simulink model "P702_NI_SoftECU"  (R2019a)
settings: Solver=ode1  StartTime=0.0  StopTime=Inf  FixedStep=0.001  RelTol=1e-3  EnableMultiTasking=on
PreLoadFcn:
  | run '.\VeriStand_BlockSet\NIVeriStandAddPaths.m'
undefined symbols (not defined in the file or in its folder): magnitude
libraries: simulink x83, simulink_extras x1
(part 44 of 76)

== system P702_NI_SoftECU/Input/GWM-SCCM//PDB//RCM//GSM/Other_GWMTx/ActiveFrontStrg_Stat_FD1 ==
  Bus_Sig : BusCreator  Inputs=5
  Counter Limited1 : simulink/Sources/Counter Limited  uplimit=15  tsamp=0.01
  Data Type Conversion1 : DataTypeConversion  OutDataTypeStr=uint8
  SteWhlBrkAnActl_No_Cnt : S-Function  Priority=1  Commented=on  FunctionName=NIVeriStandIO  Parameters=width dtype portnum stime stype btype  SFunctionDeploymentMode=off  EnableBusSupport=off  mask(NI VeriStand Inport){portnum=1, width=-1, stime=-1, dtype=auto, stype=auto, btype=1}
      mask prompts: portnum "Port number:"; width "Port dimensions (-1 for dynamically sized):"; stime "Sample time (-1 for inherited):"; dtype "Data type:"; stype "Signal type:"; btype "Block type:"
      mask help: Use this inport on any level of nested subsystems to allow NI VeriStand software to map signals to it.
      mask init:
      | NIVeriStandIO_init;
      settings: CopyFcn=NIVeriStand_MDL_functions('', 'IO_copy');  DeleteFcn=NIVeriStand_MDL_functions('', 'IO_delete');  MoveFcn=set_param(gcb, 'Mask', 'on');
      mask Callback portnum: NIVeriStand_MDL_functions('', 'IO_setportnum');
      mask TypeOptions dtype: auto | double | single | int8 | uint8 | int16 | uint16 | int32 | uint32 | boolean
      mask Callback dtype: NIVeriStand_MDL_functions('', 'IO_booleansignal');
      mask TypeOptions stype: auto | real | complex
      mask Display:
      | patch([-x x], [-y y], [.90980 .81960 .32156]);
      | plot([xrad -x x xrad], [yrad -y y yrad]);
      | fprintf('NI In%d', portnum);
  SteWhlBrkAnActl_No_Cnt_old_Debug : S-Function  Priority=1  FunctionName=NIVeriStandIO  Parameters=width dtype portnum stime stype btype  SFunctionDeploymentMode=off  EnableBusSupport=off  mask(NI VeriStand Outport){portnum=1, width=-1, stime=-1, dtype=auto, stype=auto, btype=0}
      mask prompts: portnum "Port number:"; width "Port dimensions (-1 for dynamically sized):"; stime "Sample time (-1 for inherited):"; dtype "Data type:"; stype "Signal type:"; btype "Block type:"
      mask help: Use this outport on any level of nested subsystems to allow NI VeriStand software to map signals to it.
      mask init:
      | NIVeriStandIO_init;
      settings: CopyFcn=NIVeriStand_MDL_functions('', 'IO_copy');  DeleteFcn=NIVeriStand_MDL_functions('', 'IO_delete');  MoveFcn=set_param(gcb, 'Mask', 'on');
      mask Callback portnum: NIVeriStand_MDL_functions('', 'IO_setportnum');
      mask TypeOptions dtype: auto | double | single | int8 | uint8 | int16 | uint16 | int32 | uint32 | boolean
      mask Callback dtype: NIVeriStand_MDL_functions('', 'IO_booleansignal');
      mask TypeOptions stype: auto | real | complex
      mask Display:
      | patch([-x x], [-y y], [.90980 .81960 .32156]);
      | plot([xrad -x x xrad], [yrad -y y yrad]);
      | fprintf('NI Out%d', portnum);
  SteWhlBrkAnActl_No_Cs : S-Function  Priority=1  FunctionName=NIVeriStandIO  Parameters=width dtype portnum stime stype btype  SFunctionDeploymentMode=off  EnableBusSupport=off  mask(NI VeriStand Inport){portnum=1, width=-1, stime=-1, dtype=auto, stype=auto, btype=1}
      mask prompts: portnum "Port number:"; width "Port dimensions (-1 for dynamically sized):"; stime "Sample time (-1 for inherited):"; dtype "Data type:"; stype "Signal type:"; btype "Block type:"
      mask help: Use this inport on any level of nested subsystems to allow NI VeriStand software to map signals to it.
      mask init:
      | NIVeriStandIO_init;
      settings: CopyFcn=NIVeriStand_MDL_functions('', 'IO_copy');  DeleteFcn=NIVeriStand_MDL_functions('', 'IO_delete');  MoveFcn=set_param(gcb, 'Mask', 'on');
      mask Callback portnum: NIVeriStand_MDL_functions('', 'IO_setportnum');
      mask TypeOptions dtype: auto | double | single | int8 | uint8 | int16 | uint16 | int32 | uint32 | boolean
      mask Callback dtype: NIVeriStand_MDL_functions('', 'IO_booleansignal');
      mask TypeOptions stype: auto | real | complex
      mask Display:
      | patch([-x x], [-y y], [.90980 .81960 .32156]);
      | plot([xrad -x x xrad], [yrad -y y yrad]);
      | fprintf('NI In%d', portnum);
  SteWhlBrkOffst_An_Actl : S-Function  Priority=2  FunctionName=NIVeriStandIO  Parameters=width dtype portnum stime stype btype  SFunctionDeploymentMode=off  EnableBusSupport=off  mask(NI VeriStand Inport){portnum=2, width=-1, stime=-1, dtype=auto, stype=auto, btype=1}
      mask prompts: portnum "Port number:"; width "Port dimensions (-1 for dynamically sized):"; stime "Sample time (-1 for inherited):"; dtype "Data type:"; stype "Signal type:"; btype "Block type:"
      mask help: Use this inport on any level of nested subsystems to allow NI VeriStand software to map signals to it.
      mask init:
      | NIVeriStandIO_init;
      settings: CopyFcn=NIVeriStand_MDL_functions('', 'IO_copy');  DeleteFcn=NIVeriStand_MDL_functions('', 'IO_delete');  MoveFcn=set_param(gcb, 'Mask', 'on');
      mask Callback portnum: NIVeriStand_MDL_functions('', 'IO_setportnum');
      mask TypeOptions dtype: auto | double | single | int8 | uint8 | int16 | uint16 | int32 | uint32 | boolean
      mask Callback dtype: NIVeriStand_MDL_functions('', 'IO_booleansignal');
      mask TypeOptions stype: auto | real | complex
      mask Display:
      | patch([-x x], [-y y], [.90980 .81960 .32156]);
      | plot([xrad -x x xrad], [yrad -y y yrad]);
      | fprintf('NI In%d', portnum);
  SteWhlOffstRq_D_Stat : S-Function  Priority=3  FunctionName=NIVeriStandIO  Parameters=width dtype portnum stime stype btype  SFunctionDeploymentMode=off  EnableBusSupport=off  mask(NI VeriStand Inport){portnum=3, width=-1, stime=-1, dtype=auto, stype=auto, btype=1}
      mask prompts: portnum "Port number:"; width "Port dimensions (-1 for dynamically sized):"; stime "Sample time (-1 for inherited):"; dtype "Data type:"; stype "Signal type:"; btype "Block type:"
      mask help: Use this inport on any level of nested subsystems to allow NI VeriStand software to map signals to it.
      mask init:
      | NIVeriStandIO_init;
      settings: CopyFcn=NIVeriStand_MDL_functions('', 'IO_copy');  DeleteFcn=NIVeriStand_MDL_functions('', 'IO_delete');  MoveFcn=set_param(gcb, 'Mask', 'on');
      mask Callback portnum: NIVeriStand_MDL_functions('', 'IO_setportnum');
      mask TypeOptions dtype: auto | double | single | int8 | uint8 | int16 | uint16 | int32 | uint32 | boolean
      mask Callback dtype: NIVeriStand_MDL_functions('', 'IO_booleansignal');
      mask TypeOptions stype: auto | real | complex
      mask Display:
      | patch([-x x], [-y y], [.90980 .81960 .32156]);
      | plot([xrad -x x xrad], [yrad -y y yrad]);
      | fprintf('NI In%d', portnum);
  SteWhlOffst_An_TotActl : S-Function  Priority=4  FunctionName=NIVeriStandIO  Parameters=width dtype portnum stime stype btype  SFunctionDeploymentMode=off  EnableBusSupport=off  mask(NI VeriStand Inport){portnum=4, width=-1, stime=-1, dtype=auto, stype=auto, btype=1}
      mask prompts: portnum "Port number:"; width "Port dimensions (-1 for dynamically sized):"; stime "Sample time (-1 for inherited):"; dtype "Data type:"; stype "Signal type:"; btype "Block type:"
      mask help: Use this inport on any level of nested subsystems to allow NI VeriStand software to map signals to it.
      mask init:
      | NIVeriStandIO_init;
      settings: CopyFcn=NIVeriStand_MDL_functions('', 'IO_copy');  DeleteFcn=NIVeriStand_MDL_functions('', 'IO_delete');  MoveFcn=set_param(gcb, 'Mask', 'on');
      mask Callback portnum: NIVeriStand_MDL_functions('', 'IO_setportnum');
      mask TypeOptions dtype: auto | double | single | int8 | uint8 | int16 | uint16 | int32 | uint32 | boolean
      mask Callback dtype: NIVeriStand_MDL_functions('', 'IO_booleansignal');
      mask TypeOptions stype: auto | real | complex
      mask Display:
      | patch([-x x], [-y y], [.90980 .81960 .32156]);
      | plot([xrad -x x xrad], [yrad -y y yrad]);
      | fprintf('NI In%d', portnum);
  ActiveFrontStrg_Stat_FD1_89 : Outport
  wires:
  Bus_Sig/1 -> ActiveFrontStrg_Stat_FD1_89/1  "ActiveFrontStrg_Stat_FD1_89"
  SteWhlBrkAnActl_No_Cs/1 -> Bus_Sig/2  "SteWhlBrkAnActl_No_Cs"
  SteWhlBrkOffst_An_Actl/1 -> Bus_Sig/3  "SteWhlBrkOffst_An_Actl"
  SteWhlOffstRq_D_Stat/1 -> Bus_Sig/4  "SteWhlOffstRq_D_Stat"
  SteWhlOffst_An_TotActl/1 -> Bus_Sig/5  "SteWhlOffst_An_TotActl"
  Counter Limited1/1 -> Data Type Conversion1/1
  Data Type Conversion1/1 -> SteWhlBrkAnActl_No_Cnt_old_Debug/1, Bus_Sig/1  "SteWhlBrkAnActl_No_Cnt"

== system P702_NI_SoftECU/Input/GWM-SCCM//PDB//RCM//GSM/Other_GWMTx/AllTerrainControlData_FD1 ==
  Bus_Sig : BusCreator  Inputs=4
  SelDrvMdeCnt_D_Stat : S-Function  Priority=1  FunctionName=NIVeriStandIO  Parameters=width dtype portnum stime stype btype  SFunctionDeploymentMode=off  EnableBusSupport=off  mask(NI VeriStand Inport){portnum=1, width=-1, stime=-1, dtype=auto, stype=auto, btype=1}
      mask prompts: portnum "Port number:"; width "Port dimensions (-1 for dynamically sized):"; stime "Sample time (-1 for inherited):"; dtype "Data type:"; stype "Signal type:"; btype "Block type:"
      mask help: Use this inport on any level of nested subsystems to allow NI VeriStand software to map signals to it.
      mask init:
      | NIVeriStandIO_init;
      settings: CopyFcn=NIVeriStand_MDL_functions('', 'IO_copy');  DeleteFcn=NIVeriStand_MDL_functions('', 'IO_delete');  MoveFcn=set_param(gcb, 'Mask', 'on');
      mask Callback portnum: NIVeriStand_MDL_functions('', 'IO_setportnum');
      mask TypeOptions dtype: auto | double | single | int8 | uint8 | int16 | uint16 | int32 | uint32 | boolean
      mask Callback dtype: NIVeriStand_MDL_functions('', 'IO_booleansignal');
      mask TypeOptions stype: auto | real | complex
      mask Display:
      | patch([-x x], [-y y], [.90980 .81960 .32156]);
      | plot([xrad -x x xrad], [yrad -y y yrad]);
      | fprintf('NI In%d', portnum);
  SelDrvMdeSwtchOk_D_Stat : S-Function  Priority=2  FunctionName=NIVeriStandIO  Parameters=width dtype portnum stime stype btype  SFunctionDeploymentMode=off  EnableBusSupport=off  mask(NI VeriStand Inport){portnum=2, width=-1, stime=-1, dtype=auto, stype=auto, btype=1}
      mask prompts: portnum "Port number:"; width "Port dimensions (-1 for dynamically sized):"; stime "Sample time (-1 for inherited):"; dtype "Data type:"; stype "Signal type:"; btype "Block type:"
      mask help: Use this inport on any level of nested subsystems to allow NI VeriStand software to map signals to it.
      mask init:
      | NIVeriStandIO_init;
      settings: CopyFcn=NIVeriStand_MDL_functions('', 'IO_copy');  DeleteFcn=NIVeriStand_MDL_functions('', 'IO_delete');  MoveFcn=set_param(gcb, 'Mask', 'on');
      mask Callback portnum: NIVeriStand_MDL_functions('', 'IO_setportnum');
      mask TypeOptions dtype: auto | double | single | int8 | uint8 | int16 | uint16 | int32 | uint32 | boolean
      mask Callback dtype: NIVeriStand_MDL_functions('', 'IO_booleansignal');
      mask TypeOptions stype: auto | real | complex
      mask Display:
      | patch([-x x], [-y y], [.90980 .81960 .32156]);
      | plot([xrad -x x xrad], [yrad -y y yrad]);
      | fprintf('NI In%d', portnum);
  SelDrvMdeSwtch_D_Stat : S-Function  Priority=3  FunctionName=NIVeriStandIO  Parameters=width dtype portnum stime stype btype  SFunctionDeploymentMode=off  EnableBusSupport=off  mask(NI VeriStand Inport){portnum=3, width=-1, stime=-1, dtype=auto, stype=auto, btype=1}
      mask prompts: portnum "Port number:"; width "Port dimensions (-1 for dynamically sized):"; stime "Sample time (-1 for inherited):"; dtype "Data type:"; stype "Signal type:"; btype "Block type:"
      mask help: Use this inport on any level of nested subsystems to allow NI VeriStand software to map signals to it.
      mask init:
      | NIVeriStandIO_init;
      settings: CopyFcn=NIVeriStand_MDL_functions('', 'IO_copy');  DeleteFcn=NIVeriStand_MDL_functions('', 'IO_delete');  MoveFcn=set_param(gcb, 'Mask', 'on');
      mask Callback portnum: NIVeriStand_MDL_functions('', 'IO_setportnum');
      mask TypeOptions dtype: auto | double | single | int8 | uint8 | int16 | uint16 | int32 | uint32 | boolean
      mask Callback dtype: NIVeriStand_MDL_functions('', 'IO_booleansignal');
      mask TypeOptions stype: auto | real | complex
      mask Display:
      | patch([-x x], [-y y], [.90980 .81960 .32156]);
      | plot([xrad -x x xrad], [yrad -y y yrad]);
      | fprintf('NI In%d', portnum);
  SelDrvMdeSwtch_No_Actl : S-Function  Priority=4  FunctionName=NIVeriStandIO  Parameters=width dtype portnum stime stype btype  SFunctionDeploymentMode=off  EnableBusSupport=off  mask(NI VeriStand Inport){portnum=4, width=-1, stime=-1, dtype=auto, stype=auto, btype=1}
      mask prompts: portnum "Port number:"; width "Port dimensions (-1 for dynamically sized):"; stime "Sample time (-1 for inherited):"; dtype "Data type:"; stype "Signal type:"; btype "Block type:"
      mask help: Use this inport on any level of nested subsystems to allow NI VeriStand software to map signals to it.
      mask init:
      | NIVeriStandIO_init;
      settings: CopyFcn=NIVeriStand_MDL_functions('', 'IO_copy');  DeleteFcn=NIVeriStand_MDL_functions('', 'IO_delete');  MoveFcn=set_param(gcb, 'Mask', 'on');
      mask Callback portnum: NIVeriStand_MDL_functions('', 'IO_setportnum');
      mask TypeOptions dtype: auto | double | single | int8 | uint8 | int16 | uint16 | int32 | uint32 | boolean
      mask Callback dtype: NIVeriStand_MDL_functions('', 'IO_booleansignal');
      mask TypeOptions stype: auto | real | complex
      mask Display:
      | patch([-x x], [-y y], [.90980 .81960 .32156]);
      | plot([xrad -x x xrad], [yrad -y y yrad]);
      | fprintf('NI In%d', portnum);
  AllTerrainControlData_FD1_461 : Outport
  wires:
  Bus_Sig/1 -> AllTerrainControlData_FD1_461/1  "AllTerrainControlData_FD1_461"
  SelDrvMdeCnt_D_Stat/1 -> Bus_Sig/1  "SelDrvMdeCnt_D_Stat"
  SelDrvMdeSwtchOk_D_Stat/1 -> Bus_Sig/2  "SelDrvMdeSwtchOk_D_Stat"
  SelDrvMdeSwtch_D_Stat/1 -> Bus_Sig/3  "SelDrvMdeSwtch_D_Stat"
  SelDrvMdeSwtch_No_Actl/1 -> Bus_Sig/4  "SelDrvMdeSwtch_No_Actl"

== system P702_NI_SoftECU/Input/GWM-SCCM//PDB//RCM//GSM/Other_GWMTx/All_Terrain_Data_FD1 ==
  Bus_Sig : BusCreator  Inputs=2
  TerrMde_D_RqDrv : Constant  Value=0
  TerrStat_D_RqDsply : Constant  Value=0
  All_Terrain_Data_FD1_481 : Outport
  wires:
  Bus_Sig/1 -> All_Terrain_Data_FD1_481/1  "All_Terrain_Data_FD1_481"
  TerrMde_D_RqDrv/1 -> Bus_Sig/1  "TerrMde_D_RqDrv"
  TerrStat_D_RqDsply/1 -> Bus_Sig/2  "TerrStat_D_RqDsply"

== system P702_NI_SoftECU/Input/GWM-SCCM//PDB//RCM//GSM/Other_GWMTx/BCM_Lamp_Stat_FD1 ==
  BrkWarnInd_B_Rq : Constant  Value=0
  Brk_Fluid_Lvl_Low : Constant  Value=0
  Bus_Sig : BusCreator  Inputs=35
  Courtesy_BSave_Stat : Constant
  Courtesy_Delay_Status : Constant  Value=0
  CrnrLghtLeft_Pc_Rq : Constant  Value=0
  CrnrLghtRight_Pc_Rq : Constant  Value=0
  DayRnngLampOn_B_Stat : Constant  Value=0
  DrTgateLck_D_Stat : Constant  Value=0
  Dr_Courtesy_Light_Stat : Constant  Value=0
  HeadLampLoActv_B_Stat : Constant
  HeadLampLoFlOn_B_Stat : Constant
  HeadLampLoFrOn_B_Stat : Constant
  HeadLampLoOut_B_Stat : Constant  Value=0
  HeadLghtHiFdbck_D_Stat : Constant  Value=0
  HeadLghtHiOn_B_Stat : Constant  Value=0
  HeadLghtSwtch_D_Stat : Constant  Value=2
  Headlamp_On_Wrning_Cmd : Constant  Value=0
  HomeSafeLtChime_B_Rq : Constant  Value=0
  Illuminated_Entry_Stat : Constant  Value=0
  ImpactEvntFdbck_D_Stat : Constant  Value=0
  KeyInIgnWarn_B_Cmd : Constant  Value=0
  Park_Brake_Chime_Rqst : Constant  Value=0
  PerimeterAlarmChimeRq : Constant  Value=0
  Perimeter_Alarm_Status : Constant  Value=0
  PrkLght_D_Stat : Constant  Value=0
  PrkLightChime_B_Rq : Constant  Value=0
  PudLampDrv_D_Rq : Constant  Value=0
  PudLampPsngr_D_Rq : Constant  Value=0
  PudLamp_D_Rq : Constant  Value=0
  ReducedGuard_D_Stat : Constant  Value=0
  RvrseLghtOn_B_Stat : Constant  Value=0
  StopLghtOn_B_Stat : Constant  Value=0
  TrnNotInPrkChime_B_Rq : Constant  Value=0
  WndwGlbl_D_Cmd : Constant  Value=0
  WrlssAcsyChrgInhbt_B_Rq : Constant  Value=0
  BCM_Lamp_Stat_FD1_3C3 : Outport
  wires:
  Bus_Sig/1 -> BCM_Lamp_Stat_FD1_3C3/1  "BCM_Lamp_Stat_FD1_3C3"
  BrkWarnInd_B_Rq/1 -> Bus_Sig/1  "BrkWarnInd_B_Rq"
  Brk_Fluid_Lvl_Low/1 -> Bus_Sig/2  "Brk_Fluid_Lvl_Low"
  Courtesy_BSave_Stat/1 -> Bus_Sig/3  "Courtesy_BSave_Stat"
  Courtesy_Delay_Status/1 -> Bus_Sig/4  "Courtesy_Delay_Status"
  CrnrLghtLeft_Pc_Rq/1 -> Bus_Sig/5  "CrnrLghtLeft_Pc_Rq"
  CrnrLghtRight_Pc_Rq/1 -> Bus_Sig/6  "CrnrLghtRight_Pc_Rq"
  DayRnngLampOn_B_Stat/1 -> Bus_Sig/7  "DayRnngLampOn_B_Stat"
  DrTgateLck_D_Stat/1 -> Bus_Sig/8  "DrTgateLck_D_Stat"
  Dr_Courtesy_Light_Stat/1 -> Bus_Sig/9  "Dr_Courtesy_Light_Stat"
  HeadLampLoActv_B_Stat/1 -> Bus_Sig/10  "HeadLampLoActv_B_Stat"
  HeadLampLoFlOn_B_Stat/1 -> Bus_Sig/11  "HeadLampLoFlOn_B_Stat"
  HeadLampLoFrOn_B_Stat/1 -> Bus_Sig/12  "HeadLampLoFrOn_B_Stat"
  HeadLampLoOut_B_Stat/1 -> Bus_Sig/13  "HeadLampLoOut_B_Stat"
  HeadLghtHiFdbck_D_Stat/1 -> Bus_Sig/14  "HeadLghtHiFdbck_D_Stat"
  HeadLghtHiOn_B_Stat/1 -> Bus_Sig/15  "HeadLghtHiOn_B_Stat"
  HeadLghtSwtch_D_Stat/1 -> Bus_Sig/16  "HeadLghtSwtch_D_Stat"
  Headlamp_On_Wrning_Cmd/1 -> Bus_Sig/17  "Headlamp_On_Wrning_Cmd"
  HomeSafeLtChime_B_Rq/1 -> Bus_Sig/18  "HomeSafeLtChime_B_Rq"
  Illuminated_Entry_Stat/1 -> Bus_Sig/19  "Illuminated_Entry_Stat"
  ImpactEvntFdbck_D_Stat/1 -> Bus_Sig/20  "ImpactEvntFdbck_D_Stat"
  KeyInIgnWarn_B_Cmd/1 -> Bus_Sig/21  "KeyInIgnWarn_B_Cmd"
  Park_Brake_Chime_Rqst/1 -> Bus_Sig/22  "Park_Brake_Chime_Rqst"
  PerimeterAlarmChimeRq/1 -> Bus_Sig/23  "PerimeterAlarmChimeRq"
  Perimeter_Alarm_Status/1 -> Bus_Sig/24  "Perimeter_Alarm_Status"
  PrkLght_D_Stat/1 -> Bus_Sig/25  "PrkLght_D_Stat"
  PrkLightChime_B_Rq/1 -> Bus_Sig/26  "PrkLightChime_B_Rq"
  PudLampDrv_D_Rq/1 -> Bus_Sig/27  "PudLampDrv_D_Rq"
  PudLampPsngr_D_Rq/1 -> Bus_Sig/28  "PudLampPsngr_D_Rq"
  PudLamp_D_Rq/1 -> Bus_Sig/29  "PudLamp_D_Rq"
  ReducedGuard_D_Stat/1 -> Bus_Sig/30  "ReducedGuard_D_Stat"
  RvrseLghtOn_B_Stat/1 -> Bus_Sig/31  "RvrseLghtOn_B_Stat"
  StopLghtOn_B_Stat/1 -> Bus_Sig/32  "StopLghtOn_B_Stat"
  TrnNotInPrkChime_B_Rq/1 -> Bus_Sig/33  "TrnNotInPrkChime_B_Rq"
  WndwGlbl_D_Cmd/1 -> Bus_Sig/34  "WndwGlbl_D_Cmd"
  WrlssAcsyChrgInhbt_B_Rq/1 -> Bus_Sig/35  "WrlssAcsyChrgInhbt_B_Rq"

== system P702_NI_SoftECU/Input/GWM-SCCM//PDB//RCM//GSM/Other_GWMTx/BatteryCharge_Data2_FD1 ==
  Bus_Sig : BusCreator  Inputs=1
  ChrgCrdLck_D_Falt : Constant  Value=0
  BatteryCharge_Data2_FD1_45E : Outport
  wires:
  Bus_Sig/1 -> BatteryCharge_Data2_FD1_45E/1  "BatteryCharge_Data2_FD1_45E"
  ChrgCrdLck_D_Falt/1 -> Bus_Sig/1  "ChrgCrdLck_D_Falt"

== system P702_NI_SoftECU/Input/GWM-SCCM//PDB//RCM//GSM/Other_GWMTx/Battery_Mgmt_24V_FD1 ==
  BattULo24Soc_Pc_Actl : Constant  Value=0
  BattULo24State_D_Qlty : Constant
  BattULo24_Ah_DeltaRide : Constant  Value=12800
  BattULo24_B_Falt : Constant  Value=0
  BattULo24_I_Actl : Constant  Value=8192
  Bus_Sig : BusCreator  Inputs=5
  Battery_Mgmt_24V_FD1_42E : Outport
  wires:
  Bus_Sig/1 -> Battery_Mgmt_24V_FD1_42E/1  "Battery_Mgmt_24V_FD1_42E"
  BattULo24Soc_Pc_Actl/1 -> Bus_Sig/1  "BattULo24Soc_Pc_Actl"
  BattULo24State_D_Qlty/1 -> Bus_Sig/2  "BattULo24State_D_Qlty"
  BattULo24_Ah_DeltaRide/1 -> Bus_Sig/3  "BattULo24_Ah_DeltaRide"
  BattULo24_B_Falt/1 -> Bus_Sig/4  "BattULo24_B_Falt"
  BattULo24_I_Actl/1 -> Bus_Sig/5  "BattULo24_I_Actl"

== system P702_NI_SoftECU/Input/GWM-SCCM//PDB//RCM//GSM/Other_GWMTx/Battery_Mgmt_2_FD1 ==
  BattULoChrg_D_Rq : Constant  Value=0
  BattULoSrvc_T_Actl : Constant  Value=0
  Batt_Crit_SoC_B : Constant  Value=0
  Batt_Lo_SoC_B : Constant  Value=0
  Bus_Sig : BusCreator  Inputs=14
  ChargeMode : Constant  Value=0
  EngStrtInhbt_B_RqBatt : Constant  Value=0
  IdleSpeedIncrease_El : Constant  Value=0
  PeriodicElLoad_B_Stat : Constant  Value=0
  PwSysULoFalt_D_Stat : Constant  Value=0
  Shed_Drain_Eng_Off_B : Constant  Value=0
  Shed_Feature_Group_ID : Constant  Value=0
  Shed_Level_Req : Constant  Value=0
  Shed_T_Eng_Off_B : Constant  Value=0
  ULoRgenTestMde_B_Rq : Constant  Value=0
  Battery_Mgmt_2_FD1_42C : Outport
  wires:
  Bus_Sig/1 -> Battery_Mgmt_2_FD1_42C/1  "Battery_Mgmt_2_FD1_42C"
  BattULoChrg_D_Rq/1 -> Bus_Sig/1  "BattULoChrg_D_Rq"
  BattULoSrvc_T_Actl/1 -> Bus_Sig/2  "BattULoSrvc_T_Actl"
  Batt_Crit_SoC_B/1 -> Bus_Sig/3  "Batt_Crit_SoC_B"
  Batt_Lo_SoC_B/1 -> Bus_Sig/4  "Batt_Lo_SoC_B"
  ChargeMode/1 -> Bus_Sig/5  "ChargeMode"
  EngStrtInhbt_B_RqBatt/1 -> Bus_Sig/6  "EngStrtInhbt_B_RqBatt"
  IdleSpeedIncrease_El/1 -> Bus_Sig/7  "IdleSpeedIncrease_El"
  PeriodicElLoad_B_Stat/1 -> Bus_Sig/8  "PeriodicElLoad_B_Stat"
  PwSysULoFalt_D_Stat/1 -> Bus_Sig/9  "PwSysULoFalt_D_Stat"
  Shed_Drain_Eng_Off_B/1 -> Bus_Sig/10  "Shed_Drain_Eng_Off_B"
  Shed_Feature_Group_ID/1 -> Bus_Sig/11  "Shed_Feature_Group_ID"
  Shed_Level_Req/1 -> Bus_Sig/12  "Shed_Level_Req"
  Shed_T_Eng_Off_B/1 -> Bus_Sig/13  "Shed_T_Eng_Off_B"
  ULoRgenTestMde_B_Rq/1 -> Bus_Sig/14  "ULoRgenTestMde_B_Rq"

== system P702_NI_SoftECU/Input/GWM-SCCM//PDB//RCM//GSM/Other_GWMTx/Battery_Mgmt_3_FD1 ==
  BSBattQCapAh : Constant  Value=0
  BSBattQDeltaRideAh : Constant  Value=0
  BSBattSOC : Constant  Value=0
  BSFault : Constant  Value=0
  BattULo2_Te_Actl : Constant  Value=127
  BattULoChrg_URate_RqMx : Constant  Value=5
  BattULoChrg_U_RqMn : Constant  Value=0
  BattULoChrg_U_RqMx : Constant  Value=34
  BattULoState_D_Qlty : Constant  Value=0
  Bus_Sig : BusCreator  Inputs=9
  Battery_Mgmt_3_FD1_43C : Outport
  wires:
  Bus_Sig/1 -> Battery_Mgmt_3_FD1_43C/1  "Battery_Mgmt_3_FD1_43C"
  BSBattQCapAh/1 -> Bus_Sig/1  "BSBattQCapAh"
  BSBattQDeltaRideAh/1 -> Bus_Sig/2  "BSBattQDeltaRideAh"
  BSBattSOC/1 -> Bus_Sig/3  "BSBattSOC"
  BSFault/1 -> Bus_Sig/4  "BSFault"
  BattULo2_Te_Actl/1 -> Bus_Sig/5  "BattULo2_Te_Actl"
  BattULoChrg_URate_RqMx/1 -> Bus_Sig/6  "BattULoChrg_URate_RqMx"
  BattULoChrg_U_RqMn/1 -> Bus_Sig/7  "BattULoChrg_U_RqMn"
  BattULoChrg_U_RqMx/1 -> Bus_Sig/8  "BattULoChrg_U_RqMx"
  BattULoState_D_Qlty/1 -> Bus_Sig/9  "BattULoState_D_Qlty"

== system P702_NI_SoftECU/Input/GWM-SCCM//PDB//RCM//GSM/Other_GWMTx/Battery_Mgmt_4_FD1 ==
  BattULoAuxSoc_Pc_Actl : Constant  Value=95
  BattULoAux_B_Falt : Constant  Value=0
  BattULoAux_D_Qlty : Constant  Value=0
  BattULoAux_I_Actl : Constant  Value=0
  BattULoAux_U_Actl : Constant  Value=203
  BattULoCrnkBelt_U_Pred : Constant  Value=0
  BattULoCrnkStrt_U_Pred : Constant  Value=0
  Bus_Sig : BusCreator  Inputs=7
  Battery_Mgmt_4_FD1_42B : Outport
  wires:
  Bus_Sig/1 -> Battery_Mgmt_4_FD1_42B/1  "Battery_Mgmt_4_FD1_42B"
  BattULoAuxSoc_Pc_Actl/1 -> Bus_Sig/1  "BattULoAuxSoc_Pc_Actl"
  BattULoAux_B_Falt/1 -> Bus_Sig/2  "BattULoAux_B_Falt"
  BattULoAux_D_Qlty/1 -> Bus_Sig/3  "BattULoAux_D_Qlty"
  BattULoAux_I_Actl/1 -> Bus_Sig/4  "BattULoAux_I_Actl"
  BattULoAux_U_Actl/1 -> Bus_Sig/5  "BattULoAux_U_Actl"
  BattULoCrnkBelt_U_Pred/1 -> Bus_Sig/6  "BattULoCrnkBelt_U_Pred"
  BattULoCrnkStrt_U_Pred/1 -> Bus_Sig/7  "BattULoCrnkStrt_U_Pred"

== system P702_NI_SoftECU/Input/GWM-SCCM//PDB//RCM//GSM/Other_GWMTx/Battery_Traction_1_FD1 ==
  BattTracMil_D_Rq : Constant  Value=0
  BattTracOffFst_D_Actl : Constant  Value=0
  BattTracOff_B_Actl : Constant  Value=0
  BattTrac_I_Actl : Constant  Value=0
  BattTrac_U_Actl : Constant  Value=1022
  BattTrac_U_LimHi : Constant  Value=163
  BattTrac_U_LimLo : Constant  Value=88
  Bus_Sig : BusCreator  Inputs=8
  VehStrtInhbt_B_RqBatt : Constant  Value=0
  Battery_Traction_1_FD1_7A : Outport
  wires:
  Bus_Sig/1 -> Battery_Traction_1_FD1_7A/1  "Battery_Traction_1_FD1_7A"
  BattTracMil_D_Rq/1 -> Bus_Sig/1  "BattTracMil_D_Rq"
  BattTracOffFst_D_Actl/1 -> Bus_Sig/2  "BattTracOffFst_D_Actl"
  BattTracOff_B_Actl/1 -> Bus_Sig/3  "BattTracOff_B_Actl"
  BattTrac_I_Actl/1 -> Bus_Sig/4  "BattTrac_I_Actl"
  BattTrac_U_Actl/1 -> Bus_Sig/5  "BattTrac_U_Actl"
  BattTrac_U_LimHi/1 -> Bus_Sig/6  "BattTrac_U_LimHi"
  BattTrac_U_LimLo/1 -> Bus_Sig/7  "BattTrac_U_LimLo"
  VehStrtInhbt_B_RqBatt/1 -> Bus_Sig/8  "VehStrtInhbt_B_RqBatt"

== system P702_NI_SoftECU/Input/GWM-SCCM//PDB//RCM//GSM/Other_GWMTx/Battery_Traction_3_FD1 ==
  BattTracClnt_Te_Actl : Constant  Value=164
  BattTracSoc_Pc_LimHi : Constant  Value=600
  BattTracSoc_Pc_LimLo : Constant  Value=400
  BattTracSoc_Pc_MnPrtct : Constant  Value=30
  BattTracSoc_Pc_MxPrtct : Constant  Value=700
  BattTracSrvcRqd_B_Rq : Constant  Value=0
  BattTracWarnLamp_B_Rq : Constant  Value=0
  Bus_Sig : BusCreator  Inputs=7
  Battery_Traction_3_FD1_24B : Outport
  wires:
  Bus_Sig/1 -> Battery_Traction_3_FD1_24B/1  "Battery_Traction_3_FD1_24B"
  BattTracClnt_Te_Actl/1 -> Bus_Sig/1  "BattTracClnt_Te_Actl"
  BattTracSoc_Pc_LimHi/1 -> Bus_Sig/2  "BattTracSoc_Pc_LimHi"
  BattTracSoc_Pc_LimLo/1 -> Bus_Sig/3  "BattTracSoc_Pc_LimLo"
  BattTracSoc_Pc_MnPrtct/1 -> Bus_Sig/4  "BattTracSoc_Pc_MnPrtct"
  BattTracSoc_Pc_MxPrtct/1 -> Bus_Sig/5  "BattTracSoc_Pc_MxPrtct"
  BattTracSrvcRqd_B_Rq/1 -> Bus_Sig/6  "BattTracSrvcRqd_B_Rq"
  BattTracWarnLamp_B_Rq/1 -> Bus_Sig/7  "BattTracWarnLamp_B_Rq"

== system P702_NI_SoftECU/Input/GWM-SCCM//PDB//RCM//GSM/Other_GWMTx/Battery_Traction_4_FD1 ==
  BattTracDiagClr_B_Rq : Constant  Value=0
  BattTracSoc2_Pc_Actl : Constant  Value=16382
  BattTrac_Te_Actl : Constant  Value=150
  Bus_Sig : BusCreator  Inputs=3
  Battery_Traction_4_FD1_24C : Outport
  wires:
  Bus_Sig/1 -> Battery_Traction_4_FD1_24C/1  "Battery_Traction_4_FD1_24C"
  BattTracDiagClr_B_Rq/1 -> Bus_Sig/1  "BattTracDiagClr_B_Rq"
  BattTracSoc2_Pc_Actl/1 -> Bus_Sig/2  "BattTracSoc2_Pc_Actl"
  BattTrac_Te_Actl/1 -> Bus_Sig/3  "BattTrac_Te_Actl"

== system P702_NI_SoftECU/Input/GWM-SCCM//PDB//RCM//GSM/Other_GWMTx/Battery_Traction_5_FD1 ==
  BattTrac2_Pw_ChrgInst : Constant  Value=0
  BattTrac2_Pw_DchrgInst : Constant  Value=0
  BattTrac2_Pw_LimChrg : Constant  Value=0
  BattTrac2_Pw_LimDchrg : Constant  Value=0
  Bus_Sig : BusCreator  Inputs=4
  Battery_Traction_5_FD1_24D : Outport
  wires:
  Bus_Sig/1 -> Battery_Traction_5_FD1_24D/1  "Battery_Traction_5_FD1_24D"
  BattTrac2_Pw_ChrgInst/1 -> Bus_Sig/1  "BattTrac2_Pw_ChrgInst"
  BattTrac2_Pw_DchrgInst/1 -> Bus_Sig/2  "BattTrac2_Pw_DchrgInst"
  BattTrac2_Pw_LimChrg/1 -> Bus_Sig/3  "BattTrac2_Pw_LimChrg"
  BattTrac2_Pw_LimDchrg/1 -> Bus_Sig/4  "BattTrac2_Pw_LimDchrg"

== system P702_NI_SoftECU/Input/GWM-SCCM//PDB//RCM//GSM/Other_GWMTx/Battery_Traction_6_FD1 ==
  BattTracClntPmp_D_Stat : Constant  Value=0
  BattTracCnnct_D_Cmd : Constant  Value=0
  BattTracDcdcDis_B_Rq : Constant  Value=0
  BattTracDelta_Te_Actl : Constant  Value=120
  BattTracHvilOpen_B_Stat : Constant  Value=0
  Bus_Sig : BusCreator  Inputs=6
  HtrnClntPump_D_Stat : Constant  Value=0
  Battery_Traction_6_FD1_458 : Outport
  wires:
  Bus_Sig/1 -> Battery_Traction_6_FD1_458/1  "Battery_Traction_6_FD1_458"
  BattTracClntPmp_D_Stat/1 -> Bus_Sig/1  "BattTracClntPmp_D_Stat"
  BattTracCnnct_D_Cmd/1 -> Bus_Sig/2  "BattTracCnnct_D_Cmd"
  BattTracDcdcDis_B_Rq/1 -> Bus_Sig/3  "BattTracDcdcDis_B_Rq"
  BattTracDelta_Te_Actl/1 -> Bus_Sig/4  "BattTracDelta_Te_Actl"
  BattTracHvilOpen_B_Stat/1 -> Bus_Sig/5  "BattTracHvilOpen_B_Stat"
  HtrnClntPump_D_Stat/1 -> Bus_Sig/6  "HtrnClntPump_D_Stat"

== system P702_NI_SoftECU/Input/GWM-SCCM//PDB//RCM//GSM/Other_GWMTx/BodyInfo_3_FD1 ==
  Backlit_LED_Status : Constant  Value=0
  BodySrvcRqd_B_Rq : Constant  Value=0
  Bus_Sig : BusCreator  Inputs=31
  CrashEvnt_D_Stat : Constant  Value=3
  Day_Night_Status : Constant  Value=0
  Delay_Accy : Constant  Value=0
  DimmingLvlEvnt_No_Actl : Constant  Value=0
  Dimming_Lvl : Constant  Value=12
  DrStatDrvErrCnt_B_Stat : Constant  Value=0
  DrStatDrv_B_Actl : Constant  Value=0
  DrStatHood_B_Actl : Constant  Value=0
  DrStatInnrTgate_B_Actl : Constant  Value=0
  DrStatPsngr_B_Actl : Constant  Value=0
  DrStatRl_B_Actl : Constant  Value=0
  DrStatRr_B_Actl : Constant  Value=0
  DrStatTgate_B_Actl : Constant  Value=0
  FogLghtFrontOn_B_Stat : Constant  Value=0
  FogLghtRearOn_B_Stat : Constant  Value=0
  FuelPmpInhbt_B_Stat : Constant  Value=0
  IgnKeyType_D_Actl : Constant  Value=14
  Ignition_Status : Constant  Value=0
  Key_In_Ignition_Stat : Constant  Value=0
  LifeCycMde_D_Actl : Constant  Value=0
  Litval : Constant  Value=0
  Parklamp_Status : Constant
  PrkBrkActv_B_Actl : Constant  Value=0
  Remote_Start_Status : Constant  Value=0
  TurnLghtLeftOn_B_Stat : Constant  Value=0
  TurnLghtLeft_D_Rq : Constant  Value=0
  TurnLghtRightOn_B_Stat : Constant  Value=0
  TurnLghtRight_D_Rq : Constant  Value=0
  ValetMode_D_Mem : Constant  Value=0
  BodyInfo_3_FD1_3B3 : Outport
  wires:
  Bus_Sig/1 -> BodyInfo_3_FD1_3B3/1  "BodyInfo_3_FD1_3B3"
  Backlit_LED_Status/1 -> Bus_Sig/1  "Backlit_LED_Status"
  BodySrvcRqd_B_Rq/1 -> Bus_Sig/2  "BodySrvcRqd_B_Rq"
  CrashEvnt_D_Stat/1 -> Bus_Sig/3  "CrashEvnt_D_Stat"
  Day_Night_Status/1 -> Bus_Sig/4  "Day_Night_Status"
  Delay_Accy/1 -> Bus_Sig/5  "Delay_Accy"
  DimmingLvlEvnt_No_Actl/1 -> Bus_Sig/6  "DimmingLvlEvnt_No_Actl"
  Dimming_Lvl/1 -> Bus_Sig/7  "Dimming_Lvl"
  DrStatDrvErrCnt_B_Stat/1 -> Bus_Sig/8  "DrStatDrvErrCnt_B_Stat"
  DrStatDrv_B_Actl/1 -> Bus_Sig/9  "DrStatDrv_B_Actl"
  DrStatHood_B_Actl/1 -> Bus_Sig/10  "DrStatHood_B_Actl"
  DrStatInnrTgate_B_Actl/1 -> Bus_Sig/11  "DrStatInnrTgate_B_Actl"
  DrStatPsngr_B_Actl/1 -> Bus_Sig/12  "DrStatPsngr_B_Actl"
  DrStatRl_B_Actl/1 -> Bus_Sig/13  "DrStatRl_B_Actl"
  DrStatRr_B_Actl/1 -> Bus_Sig/14  "DrStatRr_B_Actl"
  DrStatTgate_B_Actl/1 -> Bus_Sig/15  "DrStatTgate_B_Actl"
  FogLghtFrontOn_B_Stat/1 -> Bus_Sig/16  "FogLghtFrontOn_B_Stat"
  FogLghtRearOn_B_Stat/1 -> Bus_Sig/17  "FogLghtRearOn_B_Stat"
  FuelPmpInhbt_B_Stat/1 -> Bus_Sig/18  "FuelPmpInhbt_B_Stat"
  IgnKeyType_D_Actl/1 -> Bus_Sig/19  "IgnKeyType_D_Actl"
  Ignition_Status/1 -> Bus_Sig/20  "Ignition_Status"
  Key_In_Ignition_Stat/1 -> Bus_Sig/21  "Key_In_Ignition_Stat"
  LifeCycMde_D_Actl/1 -> Bus_Sig/22  "LifeCycMde_D_Actl"
  Litval/1 -> Bus_Sig/23  "Litval"
  Parklamp_Status/1 -> Bus_Sig/24  "Parklamp_Status"
  PrkBrkActv_B_Actl/1 -> Bus_Sig/25  "PrkBrkActv_B_Actl"
  Remote_Start_Status/1 -> Bus_Sig/26  "Remote_Start_Status"
  TurnLghtLeftOn_B_Stat/1 -> Bus_Sig/27  "TurnLghtLeftOn_B_Stat"
  TurnLghtLeft_D_Rq/1 -> Bus_Sig/28  "TurnLghtLeft_D_Rq"
  TurnLghtRightOn_B_Stat/1 -> Bus_Sig/29  "TurnLghtRightOn_B_Stat"
  TurnLghtRight_D_Rq/1 -> Bus_Sig/30  "TurnLghtRight_D_Rq"
  ValetMode_D_Mem/1 -> Bus_Sig/31  "ValetMode_D_Mem"

== system P702_NI_SoftECU/Input/GWM-SCCM//PDB//RCM//GSM/Other_GWMTx/Body_Info_10_FD1 ==
  Bus_Sig : BusCreator  Inputs=3
  GenericSwtch1_No_Actl : Constant  Value=0
  GenericSwtch2_No_Actl : Constant  Value=0
  GenericSwtch3_No_Actl : Constant  Value=0
  Body_Info_10_FD1_3BA : Outport
  wires:
  Bus_Sig/1 -> Body_Info_10_FD1_3BA/1  "Body_Info_10_FD1_3BA"
  GenericSwtch1_No_Actl/1 -> Bus_Sig/1  "GenericSwtch1_No_Actl"
  GenericSwtch2_No_Actl/1 -> Bus_Sig/2  "GenericSwtch2_No_Actl"
  GenericSwtch3_No_Actl/1 -> Bus_Sig/3  "GenericSwtch3_No_Actl"

== system P702_NI_SoftECU/Input/GWM-SCCM//PDB//RCM//GSM/Other_GWMTx/Body_Info_4_FD1 ==
  BattULo_I_Actl : Constant  Value=16383
  BattULo_U_Actl : Constant  Value=255
  BrkTrnShifLck_B_Stat : Constant  Value=0
  Bus_Sig : BusCreator  Inputs=15
  DcacElPw_D_Rq : Constant  Value=0
  DriverCrankingReq : Constant  Value=0
  EngOff_T_Actl : Constant  Value=0
  FuelPumpPwr_D_Stat : Constant  Value=0
  PrkLckCtlAvail_T_Stat : Constant  Value=0
  PrkLckCtlMsgTxt_D_Rq : Constant  Value=0
  PrkLckCtlTow_B_Enbl : Constant  Value=0
  PrkLckCtlUnlck_D_Stat : Constant  Value=0
  PrkLckCtl_B_Enbl : Constant  Value=0
  PtLatchActv_B_RqBcm : Constant  Value=0
  ReFuelSwtchStat_D_Actl : Constant  Value=0
  immoSecureIdleMode : Constant  Value=0
  Body_Info_4_FD1_242 : Outport
  wires:
  Bus_Sig/1 -> Body_Info_4_FD1_242/1  "Body_Info_4_FD1_242"
  BattULo_I_Actl/1 -> Bus_Sig/1  "BattULo_I_Actl"
  BattULo_U_Actl/1 -> Bus_Sig/2  "BattULo_U_Actl"
  BrkTrnShifLck_B_Stat/1 -> Bus_Sig/3  "BrkTrnShifLck_B_Stat"
  DcacElPw_D_Rq/1 -> Bus_Sig/4  "DcacElPw_D_Rq"
  DriverCrankingReq/1 -> Bus_Sig/5  "DriverCrankingReq"
  EngOff_T_Actl/1 -> Bus_Sig/6  "EngOff_T_Actl"
  FuelPumpPwr_D_Stat/1 -> Bus_Sig/7  "FuelPumpPwr_D_Stat"
  PrkLckCtlAvail_T_Stat/1 -> Bus_Sig/8  "PrkLckCtlAvail_T_Stat"
  PrkLckCtlMsgTxt_D_Rq/1 -> Bus_Sig/9  "PrkLckCtlMsgTxt_D_Rq"
  PrkLckCtlTow_B_Enbl/1 -> Bus_Sig/10  "PrkLckCtlTow_B_Enbl"
  PrkLckCtlUnlck_D_Stat/1 -> Bus_Sig/11  "PrkLckCtlUnlck_D_Stat"
  PrkLckCtl_B_Enbl/1 -> Bus_Sig/12  "PrkLckCtl_B_Enbl"
  PtLatchActv_B_RqBcm/1 -> Bus_Sig/13  "PtLatchActv_B_RqBcm"
  ReFuelSwtchStat_D_Actl/1 -> Bus_Sig/14  "ReFuelSwtchStat_D_Actl"
  immoSecureIdleMode/1 -> Bus_Sig/15  "immoSecureIdleMode"

== system P702_NI_SoftECU/Input/GWM-SCCM//PDB//RCM//GSM/Other_GWMTx/Body_Info_6_FD1 ==
  Bus_Sig : BusCreator  Inputs=15
  DrLatchMsgTxt_D_Rq : Constant  Value=0
  ElPwPoint_D_Rq : Constant  Value=0
  HeadLghtHiPrmsn_D_Stat : Constant  Value=3
  IgnPsswrdDsply_B_Rq : Constant  Value=0
  KeyAdmnTot_No_Cnt : Constant  Value=0
  KeyMykeyTot_No_Cnt : Constant  Value=0
  Keycode_Status : Constant  Value=0
  PEBackupSlot_Stats : Constant  Value=0
  PoliceIdlMde_D_Stat : Constant  Value=0
  PrmtrAlrmEvnt_D_Stat : Constant  Value=0
  PrsnlDevcChrgEnbl_B_Rq : Constant  Value=0
  SecurityMsgTxt_D_Rq : Constant  Value=0
  SteWhlLckMsgTxt_D_Rq : Constant  Value=0
  TracKeyMde_D_Stat : Constant  Value=0
  immoMsgTxt_D_Rq : Constant  Value=0
  Body_Info_6_FD1_38D : Outport
  wires:
  Bus_Sig/1 -> Body_Info_6_FD1_38D/1  "Body_Info_6_FD1_38D"
  DrLatchMsgTxt_D_Rq/1 -> Bus_Sig/1  "DrLatchMsgTxt_D_Rq"
  ElPwPoint_D_Rq/1 -> Bus_Sig/2  "ElPwPoint_D_Rq"
  HeadLghtHiPrmsn_D_Stat/1 -> Bus_Sig/3  "HeadLghtHiPrmsn_D_Stat"
  IgnPsswrdDsply_B_Rq/1 -> Bus_Sig/4  "IgnPsswrdDsply_B_Rq"
  KeyAdmnTot_No_Cnt/1 -> Bus_Sig/5  "KeyAdmnTot_No_Cnt"
  KeyMykeyTot_No_Cnt/1 -> Bus_Sig/6  "KeyMykeyTot_No_Cnt"
  Keycode_Status/1 -> Bus_Sig/7  "Keycode_Status"
  PEBackupSlot_Stats/1 -> Bus_Sig/8  "PEBackupSlot_Stats"
  PoliceIdlMde_D_Stat/1 -> Bus_Sig/9  "PoliceIdlMde_D_Stat"
  PrmtrAlrmEvnt_D_Stat/1 -> Bus_Sig/10  "PrmtrAlrmEvnt_D_Stat"
  PrsnlDevcChrgEnbl_B_Rq/1 -> Bus_Sig/11  "PrsnlDevcChrgEnbl_B_Rq"
  SecurityMsgTxt_D_Rq/1 -> Bus_Sig/12  "SecurityMsgTxt_D_Rq"
  SteWhlLckMsgTxt_D_Rq/1 -> Bus_Sig/13  "SteWhlLckMsgTxt_D_Rq"
  TracKeyMde_D_Stat/1 -> Bus_Sig/14  "TracKeyMde_D_Stat"
  immoMsgTxt_D_Rq/1 -> Bus_Sig/15  "immoMsgTxt_D_Rq"

== system P702_NI_SoftECU/Input/GWM-SCCM//PDB//RCM//GSM/Other_GWMTx/Body_Info_8_FD1 ==
  Bus_Sig : BusCreator  Inputs=7
  ChrgCordLck_B_Stat : Constant  Value=0
  ChrgCordResp1_No_Actl : Constant  Value=0
  ChrgCordResp2_No_Actl : Constant  Value=0
  WakeAlarm0_D_Stat : Constant  Value=3
  WakeAlarm1_D_Stat : Constant  Value=3
  WakeAlarm2_D_Stat : Constant  Value=3
  WakeAlarm3_D_Stat : Constant  Value=3
  Body_Info_8_FD1_3B9 : Outport
  wires:
  Bus_Sig/1 -> Body_Info_8_FD1_3B9/1  "Body_Info_8_FD1_3B9"
  ChrgCordLck_B_Stat/1 -> Bus_Sig/1  "ChrgCordLck_B_Stat"
  ChrgCordResp1_No_Actl/1 -> Bus_Sig/2  "ChrgCordResp1_No_Actl"
  ChrgCordResp2_No_Actl/1 -> Bus_Sig/3  "ChrgCordResp2_No_Actl"
  WakeAlarm0_D_Stat/1 -> Bus_Sig/4  "WakeAlarm0_D_Stat"
  WakeAlarm1_D_Stat/1 -> Bus_Sig/5  "WakeAlarm1_D_Stat"
  WakeAlarm2_D_Stat/1 -> Bus_Sig/6  "WakeAlarm2_D_Stat"
  WakeAlarm3_D_Stat/1 -> Bus_Sig/7  "WakeAlarm3_D_Stat"

== system P702_NI_SoftECU/Input/GWM-SCCM//PDB//RCM//GSM/Other_GWMTx/Body_Info_9_FD1 ==
  AdvStrt_D_Stat : Constant  Value=0
  Bus_Sig : BusCreator  Inputs=10
  CrnkInhbt_B_Stat : Constant
  CrnkInhbt_No_Cnt : Constant  Value=0
  CrnkInhbt_No_Cs : Constant  Value=0
  DrvInCtl_B_Stat : Constant  Value=0
  EngStrtActv_B_Stat : Constant  Value=0
  EngStrt_B_Rq : Constant  Value=0
  IgnPreOffActv_B_Stat : Constant  Value=0
  StrtrMtrCtlDStat_No_Cs : Constant  Value=0
  VehOnSrc_D_Stat : Constant  Value=0
  Body_Info_9_FD1_3A3 : Outport
  wires:
  Bus_Sig/1 -> Body_Info_9_FD1_3A3/1  "Body_Info_9_FD1_3A3"
  AdvStrt_D_Stat/1 -> Bus_Sig/1  "AdvStrt_D_Stat"
  CrnkInhbt_B_Stat/1 -> Bus_Sig/2  "CrnkInhbt_B_Stat"
  CrnkInhbt_No_Cnt/1 -> Bus_Sig/3  "CrnkInhbt_No_Cnt"
  CrnkInhbt_No_Cs/1 -> Bus_Sig/4  "CrnkInhbt_No_Cs"
  DrvInCtl_B_Stat/1 -> Bus_Sig/5  "DrvInCtl_B_Stat"
  EngStrtActv_B_Stat/1 -> Bus_Sig/6  "EngStrtActv_B_Stat"
  EngStrt_B_Rq/1 -> Bus_Sig/7  "EngStrt_B_Rq"
  IgnPreOffActv_B_Stat/1 -> Bus_Sig/8  "IgnPreOffActv_B_Stat"
  StrtrMtrCtlDStat_No_Cs/1 -> Bus_Sig/9  "StrtrMtrCtlDStat_No_Cs"
  VehOnSrc_D_Stat/1 -> Bus_Sig/10  "VehOnSrc_D_Stat"

== system P702_NI_SoftECU/Input/GWM-SCCM//PDB//RCM//GSM/Other_GWMTx/Climate_Cntrl_Data_2_FD1 ==
  ApaSwtch_D_RqDrv : Constant  Value=0
  ApaSwtch_No_Cnt : Constant  Value=0
  Bus_Sig : BusCreator  Inputs=12
  CabnAmb_Te_Actl : Constant  Value=0
  CamraDefog_B_Actl : Constant  Value=0
  ClimtThrmlLoad_No_Actl : Constant  Value=255
  EcoMde_D_RqDrv : Constant  Value=0
  HvacAir_Flw_Est : Constant  Value=0
  HvacBlwrFront_D_Stat : Constant  Value=0
  HvacBlwrRear_D_Stat : Constant  Value=0
  HvacRec_Pc_Est : Constant  Value=0
  HvacRemoteStrt_N_Rq : Constant  Value=0
  TwHlGrdAsst_B_RqTrn : Constant  Value=0
  Climate_Cntrl_Data_2_FD1_35E : Outport
  wires:
  Bus_Sig/1 -> Climate_Cntrl_Data_2_FD1_35E/1  "Climate_Cntrl_Data_2_FD1_35E"
  ApaSwtch_D_RqDrv/1 -> Bus_Sig/1  "ApaSwtch_D_RqDrv"
  ApaSwtch_No_Cnt/1 -> Bus_Sig/2  "ApaSwtch_No_Cnt"
  CabnAmb_Te_Actl/1 -> Bus_Sig/3  "CabnAmb_Te_Actl"
  CamraDefog_B_Actl/1 -> Bus_Sig/4  "CamraDefog_B_Actl"
  ClimtThrmlLoad_No_Actl/1 -> Bus_Sig/5  "ClimtThrmlLoad_No_Actl"
  EcoMde_D_RqDrv/1 -> Bus_Sig/6  "EcoMde_D_RqDrv"
  HvacAir_Flw_Est/1 -> Bus_Sig/7  "HvacAir_Flw_Est"
  HvacBlwrFront_D_Stat/1 -> Bus_Sig/8  "HvacBlwrFront_D_Stat"
  HvacBlwrRear_D_Stat/1 -> Bus_Sig/9  "HvacBlwrRear_D_Stat"
  HvacRec_Pc_Est/1 -> Bus_Sig/10  "HvacRec_Pc_Est"
  HvacRemoteStrt_N_Rq/1 -> Bus_Sig/11  "HvacRemoteStrt_N_Rq"
  TwHlGrdAsst_B_RqTrn/1 -> Bus_Sig/12  "TwHlGrdAsst_B_RqTrn"

== system P702_NI_SoftECU/Input/GWM-SCCM//PDB//RCM//GSM/Other_GWMTx/Climate_Control_Data_FD1 ==
  AutoHoldSwtch_D_Stat : Constant  Value=0
  Bus_Sig : BusCreator  Inputs=21
  CamraFrntBttn_D_Stat : Constant  Value=0
  CamraRearBttn_D_Stat : Constant  Value=0
  DrvSlipCtlMde_B_Rq : Constant  Value=0
  EcoInhbt_B_RqHvac : Constant  Value=0
  GlvBoxRleas_No_Actl : Constant  Value=0
  LpdbAuxBlwr_B_Rq : Constant  Value=0
  LpdbDfrstFlOn_B_Rq : Constant  Value=0
  LpdbDfrstFrOn_B_Rq : Constant  Value=0
  LpdbDfrstRearOn_B_Rq : Constant  Value=0
  LpdbHeatWiprPrk_B_Rq : Constant  Value=0
  LpdbPtc1_B_Rq : Constant  Value=0
  LpdbPtc2_B_Rq : Constant  Value=0
  LpdbPtc3_B_Rq : Constant  Value=0
  MirrorHeatOn_B_Rq : Constant  Value=0
  Outside_Air_Temp_Stat : Constant  Value=254
  PrkAidSwtch_D_RqDrv : Constant  Value=0
  PrkAidSwtch_No_Cnt : Constant  Value=0
  Remote_Start_QuietMode : Constant  Value=0
  SteWhlHeat_D_Rq : Constant  Value=0
  TrailCtlSwtch_B_Stat : Constant  Value=0
  Climate_Control_Data_FD1_41A : Outport
  wires:
  Bus_Sig/1 -> Climate_Control_Data_FD1_41A/1  "Climate_Control_Data_FD1_41A"
  AutoHoldSwtch_D_Stat/1 -> Bus_Sig/1  "AutoHoldSwtch_D_Stat"
  CamraFrntBttn_D_Stat/1 -> Bus_Sig/2  "CamraFrntBttn_D_Stat"
  CamraRearBttn_D_Stat/1 -> Bus_Sig/3  "CamraRearBttn_D_Stat"
  DrvSlipCtlMde_B_Rq/1 -> Bus_Sig/4  "DrvSlipCtlMde_B_Rq"
  EcoInhbt_B_RqHvac/1 -> Bus_Sig/5  "EcoInhbt_B_RqHvac"
  GlvBoxRleas_No_Actl/1 -> Bus_Sig/6  "GlvBoxRleas_No_Actl"
  LpdbAuxBlwr_B_Rq/1 -> Bus_Sig/7  "LpdbAuxBlwr_B_Rq"
  LpdbDfrstFlOn_B_Rq/1 -> Bus_Sig/8  "LpdbDfrstFlOn_B_Rq"
  LpdbDfrstFrOn_B_Rq/1 -> Bus_Sig/9  "LpdbDfrstFrOn_B_Rq"
  LpdbDfrstRearOn_B_Rq/1 -> Bus_Sig/10  "LpdbDfrstRearOn_B_Rq"
  LpdbHeatWiprPrk_B_Rq/1 -> Bus_Sig/11  "LpdbHeatWiprPrk_B_Rq"
  LpdbPtc1_B_Rq/1 -> Bus_Sig/12  "LpdbPtc1_B_Rq"
  LpdbPtc2_B_Rq/1 -> Bus_Sig/13  "LpdbPtc2_B_Rq"
  LpdbPtc3_B_Rq/1 -> Bus_Sig/14  "LpdbPtc3_B_Rq"
  MirrorHeatOn_B_Rq/1 -> Bus_Sig/15  "MirrorHeatOn_B_Rq"
  Outside_Air_Temp_Stat/1 -> Bus_Sig/16  "Outside_Air_Temp_Stat"
  PrkAidSwtch_D_RqDrv/1 -> Bus_Sig/17  "PrkAidSwtch_D_RqDrv"
  PrkAidSwtch_No_Cnt/1 -> Bus_Sig/18  "PrkAidSwtch_No_Cnt"
  Remote_Start_QuietMode/1 -> Bus_Sig/19  "Remote_Start_QuietMode"
  SteWhlHeat_D_Rq/1 -> Bus_Sig/20  "SteWhlHeat_D_Rq"
  TrailCtlSwtch_B_Stat/1 -> Bus_Sig/21  "TrailCtlSwtch_B_Stat"
